simulink model "Avionics"  (R2020b)
settings: Solver=VariableStepAuto  StartTime=0.0  StopTime=15  RelTol=1e-3
libraries: uavalgslib x2, sim3dcameralib x1, sim3dphyssensorlib x1, sim3dlib x1, uavsim3dlib x1, visionsinks x1, robotcorelib x1, uavutilslib x1
settings Model: EnablePacing=on  PacingRate=1000  Creator=adamm  LastModifiedBy=adamm

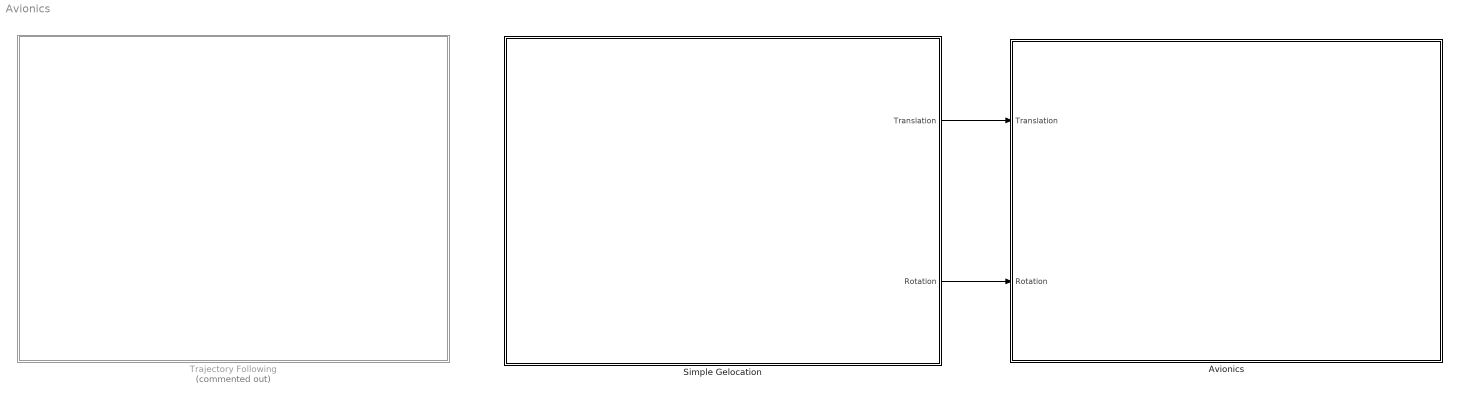
== system Avionics ==
  "Avionics " : Subsystem
  "Simple Gelocation " : Subsystem
  Trajectory Following : Subsystem  Commented=on
  wires:
  "Simple Gelocation "/1(Translation) -> "Avionics "/1(Translation)
  "Simple Gelocation "/2(Rotation) -> "Avionics "/2(Rotation)

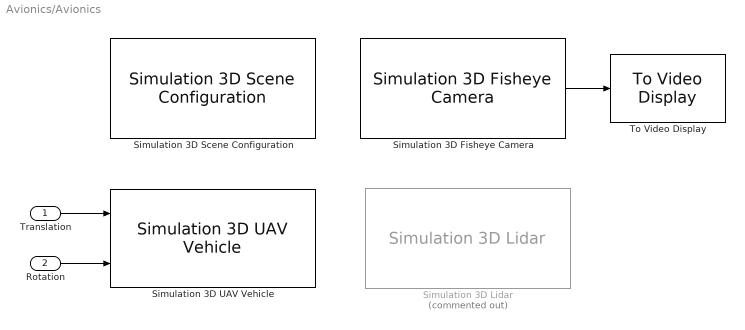
== system Avionics/Avionics  ==
  Translation : Inport
  Rotation : Inport  Port=2
  Simulation 3D Fisheye Camera : sim3dcameralib/Simulation 3D Fisheye Camera  Priority=1  sensorTag=Sim3dSensor3  sensorId=3  sensorName=Sim3dSensor3  vehTagList={'Scene Origin';'SimulinkVehicle1'}  vehTag=SimulinkVehicle1  mountLoc=Origin  offsetFlag=on  tmountOffset=[0, 0, 0]  rmountOffset=[0, 0, 0]  OpticalCenter=[640, 360]  ImageSize=[720, 1280]  RadialDistortion=[320, 0, 0, 0]  StretchMatrix=[1, 0; 0, 1]  TransformOutportEnabled=off  SampleTime=-1  mountPoint=[0 0 0]  mountOrientation=[0 0 0]  aMode=3  ID=3
      settings: SourceProductBaseCode=DR,UV,VE
  Simulation 3D Lidar : sim3dphyssensorlib/Simulation 3D Lidar  Priority=1  Commented=on  sensorTag=Sim3dSensor2  sensorId=2  sensorName=Sim3dSensor2  vehTagList={'Scene Origin';'SimulinkVehicle1'}  vehTag=SimulinkVehicle1  mountLoc=Origin  offsetFlag=on  tmountOffset=[0, 0, 0]  rmountOffset=[0, 0, 0]  DetectionRange=120  RangeResolution=0.002  VerticalFOV=40  VerticalResolution=1.25  HorizontalFOV=360  HorizontalResolution=0.16  DistanceOutportEnabled=off  TransformOutportEnabled=off  SampleTime=-1  mountPoint=[0 0 0]  mountOrientation=[0 0 0]  aMode=4  ID=2
      settings: SourceProductBaseCode=DR,UV,VE
  Simulation 3D Scene Configuration : sim3dlib/Simulation 3D Scene Configuration  Priority=0  ProjectFormat=Default Scenes  SceneDesc=US city block  ProjectName=MathWorks_Aerospace.exe  ScenePath=/Game/Maps/USCityBlock  vehTagList={'Scene Origin';'SimulinkVehicle1'}  vehTag=SimulinkVehicle1  OpVisEn=off  Ts=0.01  EnableWindow=on  sensorTag=MainCamera1  sensorId=1  sensorName=MainCamera1  mountLoc=Origin  offsetFlag=off  tmountOffset=[0, 0, 0]  rmountOffset=[0, 0, 0]  HorizontalResolution=1280  VerticalResolution=720  HorizontalFOV=60  mountPoint=[0 0 0]  mountOrientation=[0 0 0]  aMode=4  ID=1
      settings: SourceProductBaseCode=DR,UV,VE
  Simulation 3D UAV Vehicle : uavsim3dlib/Simulation 3D UAV Vehicle  Priority=-1  Mesh=Quadrotor  Color=Black  ActorName=SimulinkVehicle1  InitialTranslation=[0 0 0]  InitialRotation=[0 0 0]  SampleTime=-1  ActorType=SimulinkVehicle  ID=1  aMode=4  ActorTag=SimulinkVehicle1
      settings: SourceProductBaseCode=UV
  To Video Display : visionsinks/To Video Display  windowSizeMode=Normal  openAtMdlStart=on  fullScreen=off  videoWindowX=536805376  videoWindowY=536805376  saveWindowSize=off  videoWindowWidth=2147483647  videoWindowHeight=2147483647  inputColorFormat=RGB  inputType=Obsolete  imagePorts=One multidimensional signal  OutputDevice=On-screen video monitor  dataOrg=Column-major  isWindowOpen=off
  wires:
  Translation/1 -> Simulation 3D UAV Vehicle/1
  Rotation/1 -> Simulation 3D UAV Vehicle/2
  Simulation 3D Fisheye Camera/1 -> To Video Display/1

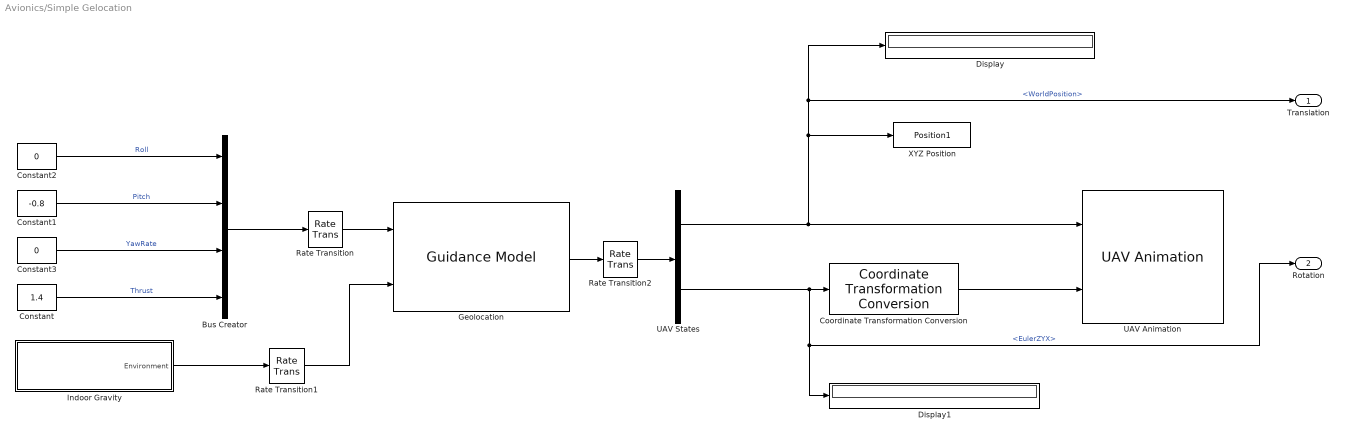
== system Avionics/Simple Gelocation  ==
  Bus Creator : BusCreator  Inputs=4  OutDataTypeStr=Bus: MultirotorGuidanceControlBus  NonVirtualBus=on
  Constant : Constant  Value=1.4
  Constant1 : Constant  Value=-0.8
  Constant2 : Constant  Value=0
  Constant3 : Constant  Value=0
  Coordinate Transformation Conversion : robotcorelib/Coordinate Transformation Conversion  InputRepresentation=Euler Angles  InputEulerSequence=ZYX  ShowTrVecInputPort=on  OutputRepresentation=Quaternion  OutputEulerSequence=ZYX  ShowTrVecOutputPort=on  SimulateUsing=Interpreted execution
      settings: SourceProductBaseCode=NV,RO,RR,UV
  Display : Display
  Display1 : Display
  "Geolocation " : uavalgslib/Guidance Model  ModelType=MultirotorGuidance  SpecifiedDataType=double  SimulateUsing=Interpreted execution  InitialWorldPositionMultirotor=[0; 0; 0]  InitialWorldVelocityMultirotor=[0; 0; 0]  InitialEulerZYXMultirotor=[0; 0; 0]  InitialBodyAngularRateRPYMultirotor=[0; 0; 0]  InitialThrustMultirotor=0  InitialNorthFixedWing=0  InitialEastFixedWing=0  InitialHeightFixedWing=0  InitialAirSpeedFixedWing=0  InitialHeadingAngleFixedWing=0  InitialFlightPathAngleFixedWing=0  InitialRollAngleFixedWing=0  InitialRollAngleRateFixedWing=0  PDRollMultirotor=[3402.97,116.67]  PDPitchMultirotor=[3402.97, 116.67]  PYawRateMultirotor=4950  PThrustMultirotor=3900  MassMultirotor=0.1  PHeightFixedWing=3.9  PHeadingAngleFixedWing=3.9  PFlightPathAngleFixedWing=39  PDRollFixedWing=[3402.97, 116.67]  PAirSpeedFixedWing=1  FlightPathAngleLimitsFixedWing=[-pi/2, pi/2]  StateBusName='MultirotorGuidanceStateBus'  ControlBusName='MultirotorGuidanceControlBus'  EnvironmentBusName='MultirotorGuidanceEnvironmentBus'  DataType=double
      settings: SourceProductBaseCode=UV
  "Indoor Gravity " : Subsystem  VariantControl=NoWind
  Rate Transition : RateTransition  Deterministic=off
  Rate Transition1 : RateTransition  Deterministic=off
  Rate Transition2 : RateTransition  Deterministic=off
  UAV Animation : uavutilslib/UAV Animation  UAVType=Multirotor  UAVSize=4  InertialZDirection=Down  SampleTime=-1
      settings: SourceProductBaseCode=UV
  UAV States : BusSelector  OutputSignals=WorldPosition,EulerZYX
  "XYZ Position " : ToWorkspace  VariableName=Position1  SaveFormat=Structure With Time  SampleTime=-1
  Translation : Outport
  Rotation : Outport  Port=2
  wires:
  "Indoor Gravity "/1(Environment) -> Rate Transition1/1
  Rate Transition1/1 -> "Geolocation "/2
  Rate Transition/1 -> "Geolocation "/1
  Rate Transition2/1 -> UAV States/1
  Constant2/1 -> Bus Creator/1  "Roll"
  UAV States/2 -> Rotation/1, Display1/1, Coordinate Transformation Conversion/1  "<EulerZYX>"
  UAV States/1 -> Translation/1, Display/1, "XYZ Position "/1, UAV Animation/1  "<WorldPosition>"
  Bus Creator/1 -> Rate Transition/1
  Constant3/1 -> Bus Creator/3  "YawRate"
  Constant/1 -> Bus Creator/4  "Thrust"
  Constant1/1 -> Bus Creator/2  "Pitch"
  "Geolocation "/1 -> Rate Transition2/1
  Coordinate Transformation Conversion/1 -> UAV Animation/2

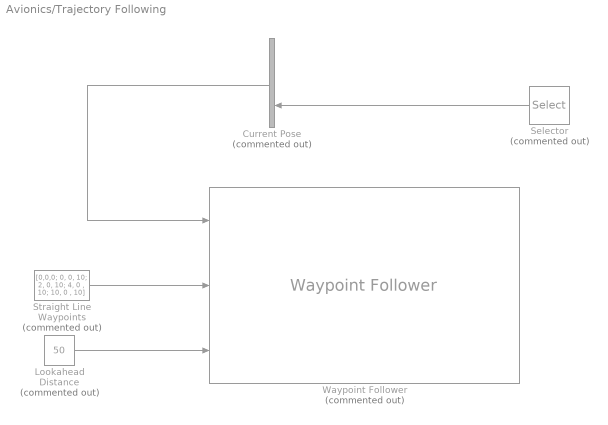
== system Avionics/Trajectory Following ==
  Current Pose : Concatenate  Commented=on
  Lookahead Distance : Constant  Commented=on  Value=50
  Selector : Selector  Commented=on  InputPortWidth=3  IndexOptions=Index vector (dialog)  Indices=[1]  OutputSizes=1
  Straight Line Waypoints : Constant  Commented=on  Value=[0,0,0; 0, 0, 10; 2, 0, 10; 4, 0 , 10; 10, 0 , 10]
  Waypoint Follower : uavalgslib/Waypoint Follower  Commented=on  UAVType=fixed-wing  StartFrom=first  TransitionRadiusSource=internal  TransitionRadius=10  MinLookaheadDistance=0.1  YawInput=off  ShowCrossTrackErrorOutput=off  ShowStatusOutput=off  SimulateUsing=Interpreted execution
      settings: SourceProductBaseCode=UV
  wires:
  Current Pose/1 -> Waypoint Follower/1
  Selector/1 -> Current Pose/2
  Straight Line Waypoints/1 -> Waypoint Follower/2
  Lookahead Distance/1 -> Waypoint Follower/3

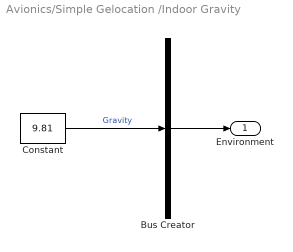
== system Avionics/Simple Gelocation /Indoor Gravity  ==
  Bus Creator : BusCreator  Inputs=1  OutDataTypeStr=Bus: MultirotorGuidanceEnvironmentBus  NonVirtualBus=on
  Constant : Constant  Value=9.81
  Environment : Outport  VectorParamsAs1DForOutWhenUnconnected=off
  wires:
  Bus Creator/1 -> Environment/1
  Constant/1 -> Bus Creator/1  "Gravity"
